simulink model "Casa_Completa"  (R2025a)
settings: Solver=ode4  StartTime=0.0  StopTime=255600  FixedStep=0.01  RelTol=1e-3
PreLoadFcn:
  | fetch_meteo;
  | setup_casa_smart;
values from neighbouring files (symbols this model uses):
  Gain_Sole_Camera = 0.6    [setup_casa_smart.m]
  Gain_Sole_Cucina = 0.6    [setup_casa_smart.m]
  Gain_Sole_Salotto = 1.0    (= 1)    [setup_casa_smart.m]
settings Model: Creator=smant  LastModifiedBy=smant
settings OptimizationCC: ZeroExternalMemoryAtStartup=off  ZeroInternalMemoryAtStartup=off
settings RTWCC: GenCodeOnly=on  TargetLang=C++
settings GRTTargetCC: TargetLangStandard=C++11 (ISO)  CodeInterfacePackaging=C++ class  SubcomponentCodeInterfacePackaging=C++ class

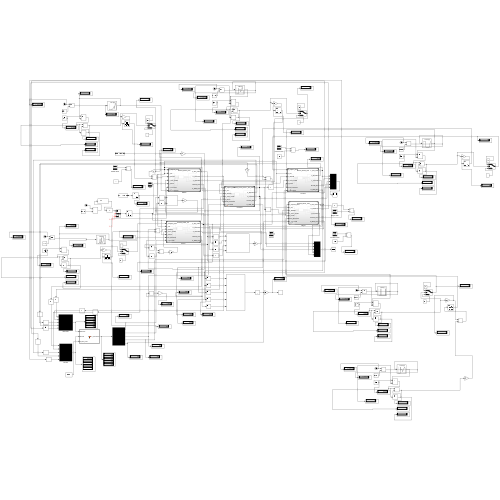
[thumbnail: Simulink's stored preview of the top-level diagram]
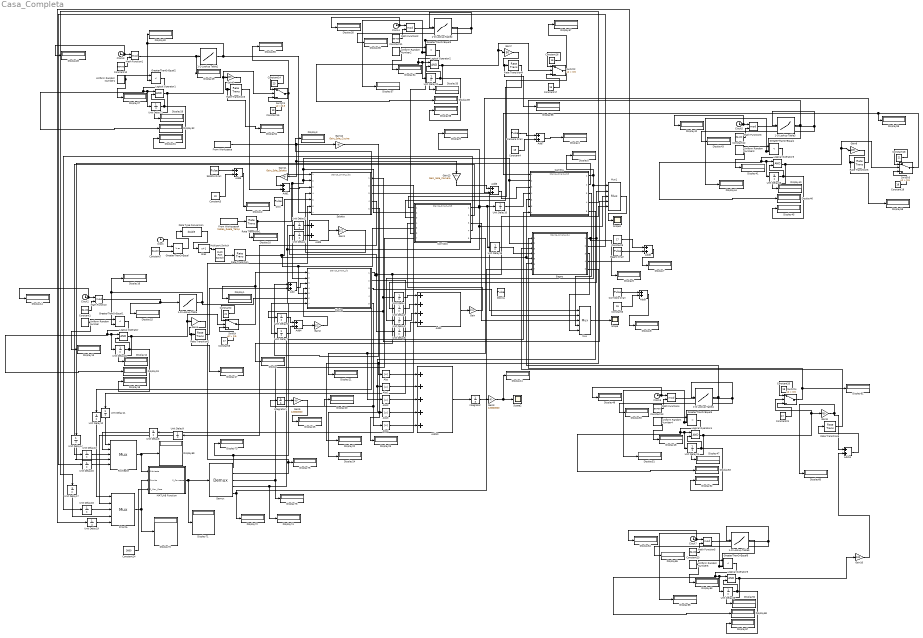
== system Casa_Completa ==
  1-D Lookup Table : Lookup_n-D  NumberOfTableDimensions=1  BreakpointsForDimension1=[0, 24000, 25200, 27000, 28800, 41500, 43200, 47000, 48600, 65000, 68400, 73000, 73800, 86400]  Table=[0, 0.1, 0.7, 0.5, 0, 0.3, 0.9, 0.7, 0.05, 0.4, 0.95, 0.8, 0, 0]  InternalRulePriority=Speed  RndMeth=Simplest
  1-D Lookup Table1 : Lookup_n-D  NumberOfTableDimensions=1  BreakpointsForDimension1=[0, 25000, 32000, 45000, 54000, 64000, 68000, 72000, 81000, 84000, 86400]  Table=[0, 0, 0.1, 0.1, 0.4, 0.5, 0.2, 0.9, 0.95, 0.5, 0]  InternalRulePriority=Speed  RndMeth=Simplest
  1-D Lookup Table2 : Lookup_n-D  NumberOfTableDimensions=1  BreakpointsForDimension1=[0, 21600, 25200, 28800, 43200, 50400, 64800, 72000, 79200, 86400]  Table=[0, 0, 0.6, 0.4, 0.5, 0.2, 0.6, 0.7, 0.3, 0]  InternalRulePriority=Speed  RndMeth=Simplest
  1-D Lookup Table3 : Lookup_n-D  NumberOfTableDimensions=1  BreakpointsForDimension1=[0, 23400, 25200, 27000, 30600, 43200, 64800, 75600, 79200, 82800, 86400]  Table=[1, 1, 0.8, 0.5, 0.1, 0.05, 0.05, 0.2, 0.7, 0.95, 1]  InternalRulePriority=Speed  RndMeth=Simplest
  1-D Lookup Table4 : Lookup_n-D  NumberOfTableDimensions=1  BreakpointsForDimension1=[0, 25140, 25200, 26400, 26460, 75540, 75600, 76800, 76860, 86400]  Table=[0, 0, 0.95, 0.95, 0, 0, 0.95, 0.95, 0, 0]  InternalRulePriority=Speed  RndMeth=Simplest
  1-D Lookup Table5 : Lookup_n-D  NumberOfTableDimensions=1  BreakpointsForDimension1=[0, 21600, 25200, 28800, 43200, 50400, 64800, 79200, 86400]  Table=[0, 0, 0.8, 0.4, 0.5, 0.2, 0.6, 0.8, 0]  InternalRulePriority=Speed  RndMeth=Simplest
  Abs{,1..4} (5 alike) : Abs  SaturateOnIntegerOverflow=off
  Add{,1,3..9,11} (10 alike) : Sum
  Add10 : Sum  Inputs=+++++
  Add2 : Sum  Inputs=++++
  Bagno : ModelReference  ModelNameDialog=Stanza_Smart_Lib4.slx  SimulationMode=Normal  ModelReferenceVersion=1.11
  Bagno Orari : DiscretePulseGenerator  Amplitude=4  Period=864000  PulseWidth=36000  PhaseDelay=234000  SampleTime=0.1
  Bias : Bias  Bias=1  SaturateOnIntegerOverflow=off
  Camera : ModelReference  ModelNameDialog=Stanza_Smart_Lib3.slx  SimulationMode=Normal  ModelReferenceVersion=1.11
  Camera Orari : DiscretePulseGenerator  Amplitude=4  Period=864000  PulseWidth=504000  PhaseDelay=324000  SampleTime=0.1
  Chill : DiscretePulseGenerator  Amplitude=300  Period=864000  PulseWidth=90000  PhaseDelay=720000  SampleTime=0.1
  Clock{,2..7} (7 alike) : Clock
  Constant{1,7,10..13,23} (7 alike) : Constant  Value=86400
  Constant14 : Constant  Value=23
  Constant15 : Constant  Value=19
  Constant16 : Constant  Value=16
  Constant17 : Constant  Value=15
  Constant18 : Constant  Value=21
  Constant19 : Constant  Value=18
  Constant2 : Constant  Value=21
  Constant20 : Constant  Value=18
  Constant21 : Constant  Value=17
  Constant24 : Constant  Value=3000
  Constant3 : Constant  Value=20
  Constant4 : Constant  Value=18
  Constant5 : Constant  Value=17
  Constant6 : Constant  Value=15
  Constant8 : Constant  Value=17
  Corridoio : ModelReference  ModelNameDialog=Stanza_Smart_Lib5.slx  SimulationMode=Normal  ModelReferenceVersion=1.11
  Corridoio Orari : DiscretePulseGenerator  Amplitude=4  Period=864000  PulseWidth=504000  PhaseDelay=648000  SampleTime=0.1
  Cucina : ModelReference  ModelNameDialog=Stanza_Smart_Lib.slx  SimulationMode=Normal  ModelReferenceVersion=1.19
  Data Type Conversion : DataTypeConversion  OutDataTypeStr=double  SaturateOnIntegerOverflow=off  RndMeth=Floor
  Demux : Demux  Outputs=5
  Display{,1..76} (77 alike) : Display
  Doccia : DiscretePulseGenerator  Amplitude=800  Period=864000  PulseWidth=12000  PhaseDelay=252000  SampleTime=0.1
  From Workspace : FromWorkspace  VariableName=Meteo_Reale_Sole  OutDataTypeStr=double  SampleTime=0.1
  From Workspace4 : FromWorkspace  VariableName=Meteo_Reale_Temp  OutputAfterFinalValue=Holding final value
  Gain : Gain  Gain=1/4
  Gain1 : Gain  Gain=1/2
  Gain10 : Gain  Gain=100  OutDataTypeStr=double
  Gain11 : Gain  Gain=Gain_Sole_Salotto
  Gain12 : Gain  Gain=Gain_Sole_Cucina
  Gain13 : Gain  Gain=Gain_Sole_Camera
  Gain2 : Gain  Gain=1/2
  Gain3 : Gain  Gain=1/3600000
  Gain4 : Gain  Gain=1500  OutDataTypeStr=double
  Gain5 : Gain  Gain=1/3600000
  Gain6 : Gain  Gain=400  OutDataTypeStr=double
  Gain7 : Gain  Gain=50  OutDataTypeStr=double
  Gain8 : Gain  Gain=100  OutDataTypeStr=double
  Gain9 : Gain  Gain=700  OutDataTypeStr=double
  GreaterThanOrEqual : RelationalOperator  OutDataTypeStr=boolean  RndMeth=Simplest  InputSameDT=off
  GreaterThanOrEqual{1..6} (6 alike) : RelationalOperator  Operator=<  OutDataTypeStr=boolean  RndMeth=Simplest  InputSameDT=off
  Integrator : Integrator
  Integrator1 : Integrator
  Logical Operator{,1..5} (6 alike) : Logic  AllPortsSameDT=off  OutDataTypeStr=boolean
  MATLAB Function : MATLAB Function  TreatAsAtomicUnit=on
  Math Function{,1..5} (6 alike) : Math  Operator=mod
  Multiport Switch : MultiPortSwitch  Inputs=2  SaturateOnIntegerOverflow=off  InputSameDT=off
  Mux : Mux  Inputs=5
  Mux1 : Mux  Inputs=5
  Priorita : Mux  Inputs=5
  Rate Transition{,1..6} (7 alike) : RateTransition  OutPortSampleTime=0.1
  Richieste : Mux  Inputs=5
  Salotto : ModelReference  ModelNameDialog=Stanza_Smart_Lib2.slx  SimulationMode=Normal  ModelReferenceVersion=1.11
  Salotto Orari : DiscretePulseGenerator  Amplitude=4  Period=864000  PulseWidth=144000  PhaseDelay=684000  SampleTime=0.1
  Scope : Scope
      settings: ActiveDisplayYMinimum=-77.809446121441937  ActiveDisplayYMaximum=78.748809567377037
  Scope1 : Scope
      settings: ActiveDisplayYMinimum=-1.4107004389747961  ActiveDisplayYMaximum=26.696303117440564
  Scope2 : Scope
      settings: ActiveDisplayYMinimum=-1  ActiveDisplayYMaximum=1  DataLoggingVariableName=ScopeData2
  Switch{,1..4} (5 alike) : Switch  Criteria=u2 > Threshold  Threshold=0.5  SaturateOnIntegerOverflow=off  InputSameDT=off
  Uniform Random Number{,1..5} (6 alike) : UniformRandomNumber  Minimum=0  Seed=42  SampleTime=300
  Unit Delay{,1..7,9..19} (19 alike) : UnitDelay  SampleTime=-1  HasFrameUpgradeWarning=on
  Unit Delay{20..25} (6 alike) : UnitDelay  SampleTime=300  HasFrameUpgradeWarning=on
  Unit Delay8 : UnitDelay  SampleTime=0.1  HasFrameUpgradeWarning=on
  wires:
  Add/1 -> Cucina/3
  Rate Transition2/1 -> Add/2
  Add1/1 -> Salotto/3
  Unit Delay/1 -> Add2/1
  Unit Delay1/1 -> Add2/2
  Unit Delay2/1 -> Add2/3
  Salotto/1 -> Display3/1, Mux1/4, Unit Delay6/1, Unit Delay/1
  Bagno/1 -> Display6/1, Mux1/2, Unit Delay1/1
  Camera/1 -> Mux1/1, Unit Delay2/1, Display5/1
  Add2/1 -> Gain/1
  Gain/1 -> Corridoio/4
  Unit Delay3/1 -> Add3/1
  Unit Delay4/1 -> Add3/2
  Cucina/1 -> Unit Delay4/1, Display/1, Mux1/5, Unit Delay5/1
  Corridoio/1 -> Unit Delay7/1, Unit Delay3/1, Mux1/3, Display9/1, Unit Delay18/1, Unit Delay10/1
  Add3/1 -> Gain1/1
  Gain1/1 -> Salotto/4
  Unit Delay6/1 -> Add4/1
  Unit Delay7/1 -> Add4/2
  Add4/1 -> Gain2/1
  Gain2/1 -> Cucina/4
  Unit Delay10/1 -> Camera/4
  Unit Delay5/1 -> Add2/4
  Salotto/3 -> Mux/1
  Cucina/3 -> Mux/2
  Corridoio/3 -> Mux/3
  Camera/3 -> Mux/4
  Bagno/3 -> Mux/5
  Mux/1 -> Scope/1
  From Workspace4/1 -> Rate Transition1/1
  Unit Delay18/1 -> Bagno/4
  Mux1/1 -> Scope1/1
  Switch/1 -> Display1/1, Cucina/1
  Constant3/1 -> Add6/2
  Salotto Orari/1 -> Add6/1
  Add6/1 -> Display2/1
  Constant4/1 -> Add7/2
  Camera Orari/1 -> Add7/1
  Add7/1 -> Display4/1
  Constant5/1 -> Add8/1
  Add8/1 -> Display7/1
  Bagno Orari/1 -> Add8/2
  Constant6/1 -> Add9/2
  Corridoio Orari/1 -> Add9/1
  Add9/1 -> Display8/1
  Multiport Switch/1 -> Rate Transition/1
  ? -> Multiport Switch/2
  ? -> Multiport Switch/3
  Clock/1 -> GreaterThanOrEqual/1
  Constant7/1 -> GreaterThanOrEqual/2
  Bias/1 -> Multiport Switch/1
  GreaterThanOrEqual/1 -> Data Type Conversion/1
  Data Type Conversion/1 -> Bias/1
  Rate Transition/1 -> Camera/5, Bagno/5, Salotto/5, Corridoio/5, Cucina/5
  Rate Transition1/1 -> Display10/1, Salotto/2, Corridoio/2, Bagno/2, Camera/2, Cucina/2
  Abs/1 -> Add10/1
  Abs1/1 -> Add10/2
  Abs2/1 -> Add10/3
  Abs3/1 -> Add10/4
  Abs4/1 -> Add10/5
  Add10/1 -> Integrator/1
  Integrator/1 -> Gain3/1
  Gain3/1 -> Scope2/1, Display11/1
  Clock2/1 -> Display14/1, Math Function/1
  Constant1/1 -> Math Function/2
  Uniform Random Number/1 -> Display13/1, GreaterThanOrEqual1/1
  Math Function/1 -> 1-D Lookup Table/1, Display15/1
  1-D Lookup Table/1 -> Cucina/6, GreaterThanOrEqual1/2, Display16/1
  Gain4/1 -> Display17/1, Rate Transition2/1
  Constant2/1 -> Switch/1
  Constant8/1 -> Switch/3
  GreaterThanOrEqual1/1 -> Logical Operator/1, Unit Delay20/1, Display19/1
  Unit Delay20/1 -> Display18/1, Logical Operator/2
  Logical Operator/1 -> Display12/1, Switch/2, Gain4/1
  From Workspace/1 -> Gain12/1, Gain13/1, Gain11/1
  Integrator1/1 -> Gain5/1
  Gain5/1 -> Display25/1
  Uniform Random Number1/1 -> Display27/1, GreaterThanOrEqual2/1
  GreaterThanOrEqual2/1 -> Logical Operator1/1, Unit Delay21/1, Display32/1
  1-D Lookup Table1/1 -> Salotto/7, GreaterThanOrEqual2/2, Display30/1
  Clock3/1 -> Display28/1, Math Function1/1
  Math Function1/1 -> 1-D Lookup Table1/1, Display29/1
  Unit Delay21/1 -> Display31/1, Logical Operator1/2
  Constant10/1 -> Math Function1/2
  Logical Operator1/1 -> Display26/1, Switch1/2, Gain6/1
  Uniform Random Number2/1 -> Display34/1, GreaterThanOrEqual3/1
  GreaterThanOrEqual3/1 -> Logical Operator2/1, Unit Delay22/1, Display39/1
  1-D Lookup Table2/1 -> Corridoio/6, Display37/1, GreaterThanOrEqual3/2
  Clock4/1 -> Display35/1, Math Function2/1
  Math Function2/1 -> 1-D Lookup Table2/1, Display36/1
  Unit Delay22/1 -> Display38/1, Logical Operator2/2
  Constant11/1 -> Math Function2/2
  Logical Operator2/1 -> Display33/1, Switch2/2, Gain7/1
  Uniform Random Number3/1 -> Display41/1, GreaterThanOrEqual4/1
  GreaterThanOrEqual4/1 -> Logical Operator3/1, Unit Delay23/1, Display46/1
  1-D Lookup Table3/1 -> Display44/1, GreaterThanOrEqual4/2, Camera/6
  Clock5/1 -> Display42/1, Math Function3/1
  Math Function3/1 -> 1-D Lookup Table3/1, Display43/1
  Unit Delay23/1 -> Display45/1, Logical Operator3/2
  Constant12/1 -> Math Function3/2
  Logical Operator3/1 -> Display40/1, Switch3/2, Gain8/1
  Uniform Random Number4/1 -> Display48/1, GreaterThanOrEqual5/1
  GreaterThanOrEqual5/1 -> Logical Operator4/1, Unit Delay24/1, Display53/1
  1-D Lookup Table4/1 -> Display51/1, GreaterThanOrEqual5/2, Bagno/6
  Clock6/1 -> Display49/1, Math Function4/1
  Math Function4/1 -> 1-D Lookup Table4/1, Display50/1
  Unit Delay24/1 -> Display52/1, Logical Operator4/2
  Constant13/1 -> Math Function4/2
  Logical Operator4/1 -> Display47/1, Switch4/2, Gain9/1
  Gain6/1 -> Display54/1, Rate Transition3/1
  Gain7/1 -> Display56/1, Rate Transition4/1
  Gain8/1 -> Display58/1, Rate Transition5/1
  Gain9/1 -> Add11/1, Display60/1
  Constant15/1 -> Switch1/3
  Constant14/1 -> Switch1/1
  Constant17/1 -> Switch2/3
  Constant16/1 -> Switch2/1
  Constant19/1 -> Switch3/3
  Constant18/1 -> Switch3/1
  Constant21/1 -> Switch4/3
  Constant20/1 -> Switch4/1
  Switch1/1 -> Display55/1, Salotto/1
  Switch2/1 -> Display57/1, Corridoio/1
  Switch3/1 -> Display59/1, Camera/1
  Switch4/1 -> Bagno/1, Display61/1
  Rate Transition3/1 -> Add1/2
  Rate Transition4/1 -> Corridoio/3
  Add5/1 -> Camera/3
  Rate Transition5/1 -> Add5/2
  Rate Transition6/1 -> Bagno/3
  Unit Delay25/1 -> Display67/1, Logical Operator5/2
  Math Function5/1 -> 1-D Lookup Table5/1, Display65/1
  Logical Operator5/1 -> Display62/1, Gain10/1
  Constant23/1 -> Math Function5/2
  1-D Lookup Table5/1 -> Display66/1, GreaterThanOrEqual6/2
  Uniform Random Number5/1 -> Display63/1, GreaterThanOrEqual6/1
  Clock7/1 -> Display64/1, Math Function5/1
  GreaterThanOrEqual6/1 -> Logical Operator5/1, Unit Delay25/1, Display68/1
  Add11/1 -> Rate Transition6/1
  Gain10/1 -> Add11/2
  Cucina/5 -> Integrator1/1, Abs4/1, Display20/1
  Salotto/5 -> Display23/1, Abs3/1
  Corridoio/5 -> Abs2/1, Display21/1
  Camera/5 -> Display24/1, Abs1/1
  Bagno/5 -> Abs/1, Display22/1
  Richieste/1 -> MATLAB Function/1(Richieste), Display69/1
  Priorita/1 -> MATLAB Function/2(Priorita), Display70/1
  MATLAB Function/1(P_Concessa) -> Display71/1, Demux/1
  Cucina/2 -> Unit Delay11/1
  Salotto/2 -> Unit Delay8/1
  Corridoio/2 -> Unit Delay13/1
  Camera/2 -> Unit Delay14/1
  Bagno/2 -> Unit Delay15/1
  Cucina/4 -> Unit Delay12/1
  Demux/1 -> Cucina/7, Display73/1
  Demux/2 -> Salotto/6, Display75/1
  Demux/3 -> Corridoio/7, Display76/1
  Demux/4 -> Camera/7, Display74/1
  Demux/5 -> Display72/1, Bagno/7
  Constant24/1 -> MATLAB Function/3(P_Max_Casa)
  Unit Delay8/1 -> Richieste/2
  Unit Delay9/1 -> Priorita/2
  Unit Delay11/1 -> Richieste/1
  Unit Delay12/1 -> Priorita/1
  Unit Delay13/1 -> Richieste/3
  Unit Delay14/1 -> Richieste/4
  Unit Delay15/1 -> Richieste/5
  Unit Delay16/1 -> Priorita/3
  Unit Delay17/1 -> Priorita/4
  Unit Delay19/1 -> Priorita/5
  Salotto/4 -> Unit Delay9/1
  Bagno/4 -> Unit Delay19/1
  Corridoio/4 -> Unit Delay16/1
  Camera/4 -> Unit Delay17/1
  Gain11/1 -> Add1/1
  Gain12/1 -> Add/1
  Gain13/1 -> Add5/1

== matlab function Casa_Completa/MATLAB Function ==
  settings: updateMethod=DISCRETE  sampleTime=0.1
  data: Richieste input; P_Concessa output; Priorita input; P_Max_Casa input
function P_Concessa = fcn(Richieste, Priorita, P_Max_Casa)
%#codegen
% GESTORE CARICHI (Resource Allocator)
% Decide chi può accendersi in base alla priorità e al limite del contatore.

N = 5; % Numero di stanze nel sistema
P_Concessa = zeros(N, 1); % Vettore di uscita inizializzato a 0
Potenza_Rimasta = P_Max_Casa;

% --- 1. PREPARAZIONE DATI ---
% Creiamo una matrice temporanea con 3 colonne:
% Col 1: Indice originale della stanza (1=Salotto, 2=Cucina, etc.)
% Col 2: La Priorità (Probabilità) di quella stanza
% Col 3: La Richiesta in Watt (Valore Assoluto, perché consumiamo sia per caldo che per freddo)
Data = zeros(N, 3);

for i = 1:N
    Data(i, 1) = i;
    Data(i, 2) = Priorita(i);
    Data(i, 3) = abs(Richieste(i)); 
end

% --- 2. CLASSIFICA (Sorting) ---
% Ordiniamo le stanze dalla priorità più alta alla più bassa.
% sort_idx conterrà gli indici ordinati (es. [2, 1, 5, 3, 4] se la cucina vince).
[~, sort_idx] = sort(Data(:, 2), 'descend');

% --- 3. ALLOCAZIONE RISORSE ---
% Scorriamo la classifica dal primo all'ultimo.
for k = 1:N
    % Chi è il k-esimo in classifica? Recuperiamo il suo indice vero.
    idx_reale = sort_idx(k);
    
    % Quanto ha chiesto questa stanza?
    watt_necessari = Data(idx_reale, 3);
    
    % Decidiamo quanto dare
    if Potenza_Rimasta >= watt_necessari
        % C'è spazio: GLIELO DIAMO TUTTO
        concessione = watt_necessari;
        Potenza_Rimasta = Potenza_Rimasta - watt_necessari;
    else
        % Non c'è abbastanza spazio: GLI DIAMO GLI AVANZI
        concessione = Potenza_Rimasta;
        Potenza_Rimasta = 0; % Contatore saturo
    end
    
    % Scriviamo il risultato nel vettore di uscita alla posizione corretta
    P_Concessa(idx_reale) = concessione;
end
